simulink model "Engine_TestBench1"  (R2017a)
settings: Solver=ode1  StartTime=0.0  StopTime=1800  FixedStep=0.01  RelTol=1e-3  EnableMultiTasking=on
PostLoadFcn:
  | , if any(exist('dsrtsu_mdlpostloadfcn', 'file') == [2, 3, 6]), try dsrtsu_mdlpostloadfcn('Execute', bdroot); catch fprintf('Error in PostLoadFcn (dsrtsu_mdlpostloadfcn) for model "%s":\n %s\n', bdroot, lasterr); end, end,
undefined symbols (not defined in the file): air, Engine, env, max_vehicle_rad_air_flow, NeutralGear, ParkGear
libraries: simulink x19, EC2_libraries x2
(part 2 of 2)

== system Engine_TestBench1/ICE Simple/Engine Plant Modified/Core Engine/Crank Process/function ==
  EngSpd : Inport
  f : TriggerPort  TriggerType=function-call  VariantControl=Variant
      settings: CopyFcn=Stateflow.SLINSF.SimulinkMan.removeBlockPreDeleteFcn  PreDeleteFcn=Stateflow.SLINSF.SimulinkMan.unsafePredeleteFcn
  1-D Lookup Table : Lookup_n-D  NumberOfTableDimensions=1  BreakpointsForDimension1=[0 50 120 210 300 320 340 350 400]  Table=[90 90 90 90 90 90 90 90 90]  InternalRulePriority=Speed  RndMeth=Simplest  InputSameDT=on
  Sine Wave : Sin  Amplitude=20  Frequency=41.88
  Sum : Sum
  CrankTrq : Outport
  wires:
  1-D Lookup Table/1 -> Sum/1
  EngSpd/1 -> 1-D Lookup Table/1
  Sum/1 -> CrankTrq/1
  Sine Wave/1 -> Sum/2

== system Engine_TestBench1/ICE Simple/Engine Plant Modified/Core Engine/EngEfficiency ==
  note: Mechanical Power [W]
  Torque : Inport
  Speed : Inport  Port=2
  Fuel Consumption : Inport  Port=3
  Divide by Zero Fix : Subsystem
  Divide_by_Zero_Fix1 : EC2_libraries/Divide_by_Zero_Fix  Commented=on
  From1 : From  Commented=on  GotoTag=Wh_out
  From2 : From  Commented=on  GotoTag=Wh_in
  Goto1 : Goto  Commented=on  GotoTag=Wh_out
  Goto2 : Goto  Commented=on  GotoTag=Wh_in
  Integrator1 : Integrator  Commented=on  LimitOutput=on  LowerSaturationLimit=0
  Integrator2 : Integrator  Commented=on  LimitOutput=on  LowerSaturationLimit=0
  OnlyPositiveEnergy : Saturate  Commented=on  UpperLimit=inf  LowerLimit=0
  Percentage Efficiency : Gain  Gain=100
  Product : Product  RndMeth=Zero
  "RPM to rad/s " : Gain  Gain=pi/30
  Scope : Scope  NumInputPorts=2
  Specific Energy LHV in J/kg : Gain  Gain=Engine.Fuel.Lower_Heating_Value/1000
  Sum : Sum  Inputs=-+
  To Workspace7 : ToWorkspace  Commented=on  VariableName=eng_Wh_pos_eff_hist  SampleTime=-1
      settings: Decimation=WORKSPACE_DECIMATION
  engine_efficiency : Scope
  limit_efficiency[0-100%] : Saturate  UpperLimit=100  LowerLimit=0  ZeroCross=off
  PowerLoss : Outport
  wires:
  limit_efficiency[0-100%]/1 -> engine_efficiency/1
  Sum/1 -> PowerLoss/1  "Losses [W]"
  Fuel Consumption/1 -> Specific Energy LHV in J/kg/1
  Specific Energy LHV in J/kg/1 -> Divide by Zero Fix/2(Divide), Sum/2, Integrator2/1, Scope/2  "Thermal Power [W]"
  Torque/1 -> Product/2  "Nm"
  Speed/1 -> "RPM to rad/s "/1  "rpm"
  Percentage Efficiency/1 -> limit_efficiency[0-100%]/1  "Efficiency [%]"
  Divide by Zero Fix/1(Output) -> Percentage Efficiency/1
  Product/1 -> Scope/1, Divide by Zero Fix/1(Multiply), OnlyPositiveEnergy/1, Sum/1  "wer [W]"
  Divide_by_Zero_Fix1/1 -> To Workspace7/1
  From1/1 -> Divide_by_Zero_Fix1/1
  From2/1 -> Divide_by_Zero_Fix1/2
  Integrator1/1 -> Goto1/1
  OnlyPositiveEnergy/1 -> Integrator1/1
  Integrator2/1 -> Goto2/1
  "RPM to rad/s "/1 -> Product/1

== system Engine_TestBench1/ICE Simple/Engine Plant Modified/Core Engine/EngineThermal ==
  note: Temp Delta C deg
  PowerLoss : Inport
  Divide : Product  Inputs=*/
  Divide1 : Product  Inputs=**
  Engine Mass : Constant  Value=Engine.Mass
  Memory : Memory  X0=Engine.Init_T_amb
  Memory1 : Memory
  Product : Product  RndMeth=Zero
  Specific Heat Cap Aluminum : Constant  Value=Engine.Specific_Heat
  Sum : Sum  Inputs=|++
  Sum1 : Sum  Inputs=|+-
  tloop : Constant  Value=0.01
  Temp[degC] : Outport
  tag scope: Heat_Transfer_Eng_1=global
  wires:
  Memory1/1 -> Sum1/2
  Divide1/1 -> Divide/1  "J"
  Sum1/1 -> Divide1/2
  Memory/1 -> Sum/2
  PowerLoss/1 -> Sum1/1, [Heat_Transfer_Eng_1]  "J/s"
  Engine Mass/1 -> Product/1  "kg"
  Specific Heat Cap Aluminum/1 -> Product/2  "J/kg*K"
  Product/1 -> Divide/2
  Sum/1 -> Memory/1, Temp[degC]/1
  Divide/1 -> Sum/1
  tloop/1 -> Divide1/1
  [Heat_Reject_Eng] -> Memory1/1

== system Engine_TestBench1/ICE Simple/Engine Plant Modified/Radiator/Divide by Zero Fix ==
  Multiply : Inport
  Divide : Inport  Port=2
  Compare To Zero : simulink/Logic and Bit Operations/Compare To Zero  relop=<=  OutDataTypeStr=boolean
  Constant1 : Constant  Value=0
  Constant2 : Constant
  Product2 : Product  Inputs=/*  SaturateOnIntegerOverflow=on  InputSameDT=on  OutDataTypeStr=Inherit: Same as first input
  Switch : Switch  Threshold=1
  Switch1 : Switch  Threshold=1
  Output : Outport
  wires:
  Multiply/1 -> Product2/2
  Switch1/1 -> Output/1
  Constant1/1 -> Switch1/1
  Product2/1 -> Switch1/3
  Switch/1 -> Product2/1
  Divide/1 -> Switch/3, Compare To Zero/1
  Constant2/1 -> Switch/1
  Compare To Zero/1 -> Switch1/2, Switch/2

== system Engine_TestBench1/ICE Simple/Soft ECM/Fuel Consumption/Divide by Zero Fix ==
  Divide : Inport
  Multiply : Inport  Port=2
  Compare To Zero : simulink/Logic and Bit Operations/Compare To Zero  relop=<=  OutDataTypeStr=boolean
  Constant1 : Constant  Value=0
  Constant2 : Constant
  Product2 : Product  Inputs=/*  SaturateOnIntegerOverflow=on  InputSameDT=on  OutDataTypeStr=Inherit: Same as first input
  Switch : Switch  Threshold=1
  Switch1 : Switch  Threshold=1
  Output : Outport
  wires:
  Multiply/1 -> Product2/2
  Switch1/1 -> Output/1
  Constant1/1 -> Switch1/1
  Product2/1 -> Switch1/3
  Switch/1 -> Product2/1
  Divide/1 -> Compare To Zero/1, Switch/3
  Constant2/1 -> Switch/1
  Compare To Zero/1 -> Switch1/2, Switch/2

== system Engine_TestBench1/ICE Simple/Soft ECM/Fuel Consumption/Divide by Zero Fix1 ==
  Divide : Inport
  Multiply : Inport  Port=2
  Compare To Zero : simulink/Logic and Bit Operations/Compare To Zero  relop=<=  OutDataTypeStr=boolean
  Constant1 : Constant  Value=0
  Constant2 : Constant
  Product2 : Product  Inputs=/*  SaturateOnIntegerOverflow=on  InputSameDT=on  OutDataTypeStr=Inherit: Same as first input
  Switch : Switch  Threshold=1
  Switch1 : Switch  Threshold=1
  Output : Outport
  wires:
  Compare To Zero/1 -> Switch/2, Switch1/2
  Constant2/1 -> Switch/1
  Divide/1 -> Compare To Zero/1, Switch/3
  Switch/1 -> Product2/1
  Product2/1 -> Switch1/3
  Constant1/1 -> Switch1/1
  Switch1/1 -> Output/1
  Multiply/1 -> Product2/2

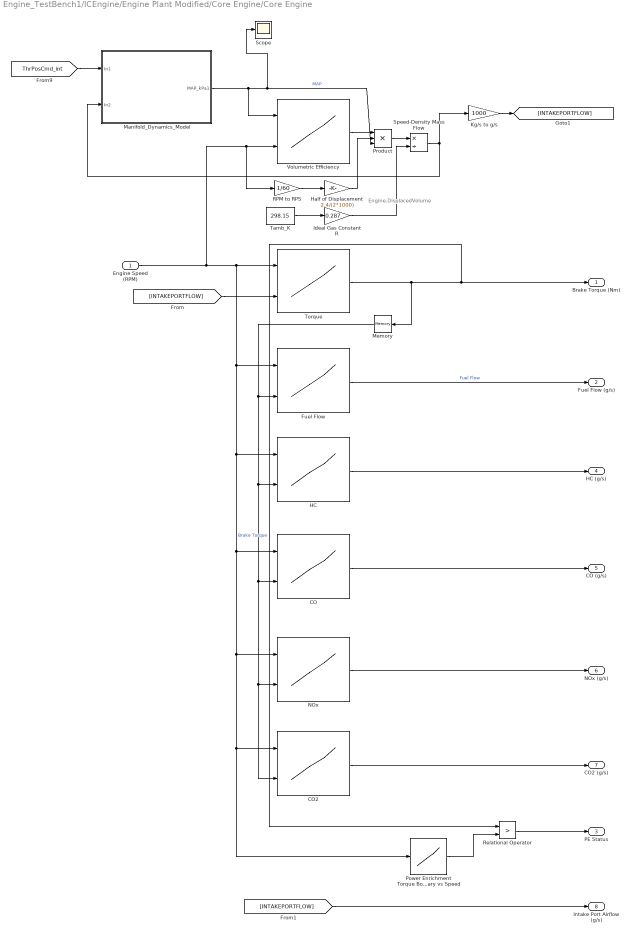
== system Engine_TestBench1/ICEngine/Engine Plant Modified/Core Engine/Core Engine ==
  note: Engine.DisplacedVolume
  Engine Speed (RPM) : Inport
  CO : Lookup2D  RowIndex=Engine.Engine.Emissions.SPEED  ColumnIndex=Engine.Engine.Emissions.TQ  Table=Engine.Engine.Emissions.CO/1000  LookUpMeth=Interpolation-Use End Values
  CO2 : Lookup2D  RowIndex=Engine.Engine.Emissions.SPEED  ColumnIndex=Engine.Engine.Emissions.TQ  Table=Engine.Engine.Emissions.CO2/1000  LookUpMeth=Interpolation-Use End Values
  Fuel Flow : Lookup2D  RowIndex=Engine.Engine.FuelFlow.SPEED  ColumnIndex=Engine.Engine.FuelFlow.TQ  Table=Engine.Engine.FuelFlow.FuelFlow  LookUpMeth=Interpolation-Use End Values
  HC : Lookup2D  RowIndex=Engine.Engine.Emissions.SPEED  ColumnIndex=Engine.Engine.Emissions.TQ  Table=Engine.Engine.Emissions.HC/1000  LookUpMeth=Interpolation-Use End Values
  Half of Displacement : Gain  Gain=2.4/(2*1000)
  Ideal Gas Constant R : Gain  Gain=0.287
  Kg/s to g/s : Gain  Gain=1000
  Manifold_Dynamics_Model : Subsystem
  Memory : Memory
  NOx : Lookup2D  RowIndex=Engine.Engine.Emissions.SPEED  ColumnIndex=Engine.Engine.Emissions.TQ  Table=Engine.Engine.Emissions.NOx/1000  LookUpMeth=Interpolation-Use End Values
  Power Enrichment Torque Boundary vs Speed : Lookup_n-D  NumberOfTableDimensions=1  BreakpointsForDimension1=Engine.Engine.PEBound.SPEED  Table=Engine.Engine.PEBound.PEBound  ExtrapMethod=Clip  InternalRulePriority=Speed  RndMeth=Simplest  InputSameDT=on
  Product : Product  Inputs=***
  RPM to RPS : Gain  Gain=1/60
  Relational Operator : RelationalOperator  Operator=>  OutDataTypeStr=boolean  RndMeth=Nearest
  Scope : Scope
  Speed-Density Mass Flow : Product  Inputs=*/
  Tamb_K : Constant  Value=298.15
  Torque : Lookup2D  RowIndex=Engine.Engine.TQ.SPEED  ColumnIndex=Engine.Engine.TQ.MAF  Table=Engine.Engine.TQ.TQ  LookUpMeth=Interpolation-Use End Values
  Volumetric Efficiency : Lookup2D  RowIndex=Engine.Engine.VE.MAP  ColumnIndex=Engine.Engine.VE.SPEED  Table=Engine.Engine.VE.VE  LookUpMeth=Interpolation-Use End Values
  Brake Torque (Nm) : Outport
  Fuel Flow (g/s) : Outport  Port=2
  PE Status : Outport  Port=3
  HC (g/s) : Outport  Port=4
  CO (g/s) : Outport  Port=5
  NOx (g/s) : Outport  Port=6
  CO2 (g/s) : Outport  Port=7
  Intake Port Airflow (g/s) : Outport  Port=8
  wires:
  Torque/1 -> Brake Torque (Nm)/1, Relational Operator/1, Memory/1  "Brake Torque"
  [INTAKEPORTFLOW] -> Torque/2
  Fuel Flow/1 -> Fuel Flow (g/s)/1  "Fuel Flow"
  Memory/1 -> CO2/2, NOx/2, CO/2, HC/2, Fuel Flow/2
  Power Enrichment Torque Boundary vs Speed/1 -> Relational Operator/2
  Relational Operator/1 -> PE Status/1
  HC/1 -> HC (g/s)/1
  CO/1 -> CO (g/s)/1
  NOx/1 -> NOx (g/s)/1
  CO2/1 -> CO2 (g/s)/1
  [INTAKEPORTFLOW] -> Intake Port Airflow (g/s)/1
  Volumetric Efficiency/1 -> Product/1
  Ideal Gas Constant R/1 -> Speed-Density Mass Flow/2
  Product/1 -> Speed-Density Mass Flow/1
  Tamb_K/1 -> Ideal Gas Constant R/1
  RPM to RPS/1 -> Half of Displacement/1
  Half of Displacement/1 -> Product/2
  Engine Speed (RPM)/1 -> Torque/1, Fuel Flow/1, HC/1, CO/1, NOx/1, Power Enrichment Torque Boundary vs Speed/1, CO2/1, RPM to RPS/1, Volumetric Efficiency/2
  [ThrPosCmd_int] -> Manifold_Dynamics_Model/1(In1)
  Manifold_Dynamics_Model/1(MAP_kPa1) -> Volumetric Efficiency/1, Scope/1, Product/3  "MAP"
  Kg/s to g/s/1 -> [INTAKEPORTFLOW]
  Speed-Density Mass Flow/1 -> Manifold_Dynamics_Model/2(In2), Kg/s to g/s/1

== system Engine_TestBench1/ICEngine/Engine Plant Modified/Core Engine/Crank Process/function ==
  EngSpd : Inport
  f : TriggerPort  TriggerType=function-call  VariantControl=Variant
      settings: CopyFcn=Stateflow.SLINSF.SimulinkMan.removeBlockPreDeleteFcn  PreDeleteFcn=Stateflow.SLINSF.SimulinkMan.unsafePredeleteFcn
  1-D Lookup Table : Lookup_n-D  NumberOfTableDimensions=1  BreakpointsForDimension1=[0 50 120 210 300 320 340 350 400]  Table=[90 90 90 90 90 90 90 90 90]  InternalRulePriority=Speed  RndMeth=Simplest  InputSameDT=on
  Sine Wave : Sin  Amplitude=20  Frequency=41.88
  Sum : Sum
  CrankTrq : Outport
  wires:
  1-D Lookup Table/1 -> Sum/1
  EngSpd/1 -> 1-D Lookup Table/1
  Sum/1 -> CrankTrq/1
  Sine Wave/1 -> Sum/2

== system Engine_TestBench1/ICEngine/Engine Plant Modified/Core Engine/EngEfficiency ==
  note: Mechanical Power [W]
  Torque : Inport
  Speed : Inport  Port=2
  Fuel Consumption : Inport  Port=3
  Divide by Zero Fix : Subsystem
  Divide_by_Zero_Fix1 : EC2_libraries/Divide_by_Zero_Fix  Commented=on
  From1 : From  Commented=on  GotoTag=Wh_out
  From2 : From  Commented=on  GotoTag=Wh_in
  Goto1 : Goto  Commented=on  GotoTag=Wh_out
  Goto2 : Goto  Commented=on  GotoTag=Wh_in
  Integrator1 : Integrator  Commented=on  LimitOutput=on  LowerSaturationLimit=0
  Integrator2 : Integrator  Commented=on  LimitOutput=on  LowerSaturationLimit=0
  OnlyPositiveEnergy : Saturate  Commented=on  UpperLimit=inf  LowerLimit=0
  Percentage Efficiency : Gain  Gain=100
  Product : Product  RndMeth=Zero
  "RPM to rad/s " : Gain  Gain=pi/30
  Scope : Scope  NumInputPorts=2
  Specific Energy LHV in J/kg : Gain  Gain=Engine.Fuel.Lower_Heating_Value/1000
  Sum : Sum  Inputs=-+
  To Workspace7 : ToWorkspace  Commented=on  VariableName=eng_Wh_pos_eff_hist  SampleTime=-1
      settings: Decimation=WORKSPACE_DECIMATION
  engine_efficiency : Scope
  limit_efficiency[0-100%] : Saturate  UpperLimit=100  LowerLimit=0
  PowerLoss : Outport
  wires:
  limit_efficiency[0-100%]/1 -> engine_efficiency/1
  Sum/1 -> PowerLoss/1  "Losses [W]"
  Fuel Consumption/1 -> Specific Energy LHV in J/kg/1
  Specific Energy LHV in J/kg/1 -> Divide by Zero Fix/2(Divide), Sum/2, Integrator2/1, Scope/2  "Thermal Power [W]"
  Torque/1 -> Product/2  "Nm"
  Speed/1 -> "RPM to rad/s "/1  "rpm"
  Percentage Efficiency/1 -> limit_efficiency[0-100%]/1  "Efficiency [%]"
  Divide by Zero Fix/1(Output) -> Percentage Efficiency/1
  Product/1 -> Scope/1, Divide by Zero Fix/1(Multiply), OnlyPositiveEnergy/1, Sum/1  "wer [W]"
  Divide_by_Zero_Fix1/1 -> To Workspace7/1
  From1/1 -> Divide_by_Zero_Fix1/1
  From2/1 -> Divide_by_Zero_Fix1/2
  Integrator1/1 -> Goto1/1
  OnlyPositiveEnergy/1 -> Integrator1/1
  Integrator2/1 -> Goto2/1
  "RPM to rad/s "/1 -> Product/1

== system Engine_TestBench1/ICEngine/Engine Plant Modified/Core Engine/EngineThermal ==
  note: Temp Delta C deg
  PowerLoss : Inport
  Divide : Product  Inputs=*/
  Divide1 : Product  Inputs=**
  Engine Mass : Constant  Value=Engine.Mass
  Memory : Memory  X0=Engine.Init_T_amb
  Memory1 : Memory
  Product : Product  RndMeth=Zero
  Specific Heat Cap Aluminum : Constant  Value=Engine.Specific_Heat
  Sum : Sum  Inputs=|++
  Sum1 : Sum  Inputs=|+-
  tloop : Constant  Value=0.01
  Temp[degC] : Outport
  tag scope: Heat_Transfer_Eng=global
  wires:
  Memory1/1 -> Sum1/2
  Divide1/1 -> Divide/1  "J"
  Sum1/1 -> Divide1/2
  Memory/1 -> Sum/2
  PowerLoss/1 -> Sum1/1, [Heat_Transfer_Eng]  "J/s"
  Engine Mass/1 -> Product/1  "kg"
  Specific Heat Cap Aluminum/1 -> Product/2  "J/kg*K"
  Product/1 -> Divide/2
  Sum/1 -> Memory/1, Temp[degC]/1
  Divide/1 -> Sum/1
  tloop/1 -> Divide1/1
  [Heat_Reject_Eng] -> Memory1/1

== system Engine_TestBench1/ICEngine/Engine Plant Modified/Radiator/Divide by Zero Fix ==
  Multiply : Inport
  Divide : Inport  Port=2
  Compare To Zero : simulink/Logic and Bit Operations/Compare To Zero  relop===  OutDataTypeStr=boolean
  Constant1 : Constant  Value=0
  Constant2 : Constant
  Product2 : Product  Inputs=/*  SaturateOnIntegerOverflow=on  InputSameDT=on  OutDataTypeStr=Inherit: Same as first input
  Switch : Switch  Threshold=1
  Switch1 : Switch  Threshold=1
  Output : Outport
  wires:
  Multiply/1 -> Product2/2
  Switch1/1 -> Output/1
  Constant1/1 -> Switch1/1
  Product2/1 -> Switch1/3
  Switch/1 -> Product2/1
  Divide/1 -> Switch/3, Compare To Zero/1
  Constant2/1 -> Switch/1
  Compare To Zero/1 -> Switch1/2, Switch/2

== system Engine_TestBench1/ICEngine/Soft ECM/Fuel Consumption/Divide by Zero Fix ==
  Divide : Inport
  Multiply : Inport  Port=2
  Compare To Zero : simulink/Logic and Bit Operations/Compare To Zero  relop===  OutDataTypeStr=boolean
  Constant1 : Constant  Value=0
  Constant2 : Constant
  Product2 : Product  Inputs=/*  SaturateOnIntegerOverflow=on  InputSameDT=on  OutDataTypeStr=Inherit: Same as first input
  Switch : Switch  Threshold=1
  Switch1 : Switch  Threshold=1
  Output : Outport
  wires:
  Multiply/1 -> Product2/2
  Switch1/1 -> Output/1
  Constant1/1 -> Switch1/1
  Product2/1 -> Switch1/3
  Switch/1 -> Product2/1
  Divide/1 -> Compare To Zero/1, Switch/3
  Constant2/1 -> Switch/1
  Compare To Zero/1 -> Switch1/2, Switch/2

== system Engine_TestBench1/ICEngine/Soft ECM/Fuel Consumption/Divide by Zero Fix1 ==
  Divide : Inport
  Multiply : Inport  Port=2
  Compare To Zero : simulink/Logic and Bit Operations/Compare To Zero  relop===  OutDataTypeStr=boolean
  Constant1 : Constant  Value=0
  Constant2 : Constant
  Product2 : Product  Inputs=/*  SaturateOnIntegerOverflow=on  InputSameDT=on  OutDataTypeStr=Inherit: Same as first input
  Switch : Switch  Threshold=1
  Switch1 : Switch  Threshold=1
  Output : Outport
  wires:
  Compare To Zero/1 -> Switch/2, Switch1/2
  Constant2/1 -> Switch/1
  Divide/1 -> Compare To Zero/1, Switch/3
  Switch/1 -> Product2/1
  Product2/1 -> Switch1/3
  Constant1/1 -> Switch1/1
  Switch1/1 -> Output/1
  Multiply/1 -> Product2/2

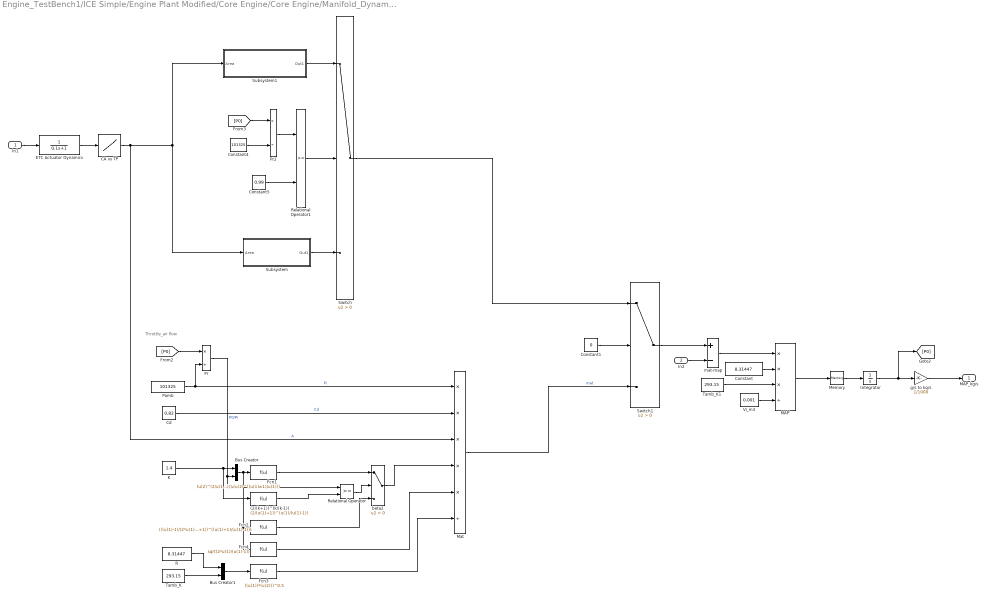
== system Engine_TestBench1/ICE Simple/Engine Plant Modified/Core Engine/Core Engine/Manifold_Dynamics_Model ==
  note: Throttle_air flow
  In1 : Inport
  In2 : Inport  Port=2
  (2/(k+1))^(k/(k-1)) : Fcn  Expr=(2/(u(1)+1))^(u(1)/(u(1)-1))
  Bus Creator : BusCreator  Inputs=2
  Bus Creator1 : BusCreator  Inputs=2
  CA vs TP : Lookup  InputValues=Engine.Throttle.CA.TPP  Table=Engine.Throttle.CA.CA  LookUpMeth=Interpolation-Use End Values
  Cd : Constant  Value=0.82
  Constant : Constant  Value=8.31447
  Constant1 : Constant  Value=0
  Constant4 : Constant  Value=101325
  Constant5 : Constant  Value=0.99
  ETC Actuator Dynamics : TransferFcn  Denominator=[0.1 1]
  Fcn1 : Fcn  Expr=(u(2)^(2/u(1)))-(u(2)^((u(1)+1)/u(1)))
  Fcn2 : Fcn  Expr=(((u(1)-1)/(2*u(1)))*(2/(u(1)+1))^((u(1)+1)/(u(1)-1)))
  Fcn3 : Fcn  Expr=((u(1))*(u(2)))^0.5
  Fcn4 : Fcn  Expr=sqrt(2*u(1)/(u(1)-1))
  Integrator : Integrator  InitialCondition=101325
  K : Constant  Value=1.4
  MAP' : Product  Inputs=***/
  Mat : Product  Inputs=*****/
  Memory : Memory
  Pamb : Constant  Value=101325
  Pr : Product  Inputs=*/
  Pr2 : Product  Inputs=*/
  R : Constant  Value=8.31447
  Relational Operator : RelationalOperator  OutDataTypeStr=boolean  ZeroCross=off  RndMeth=Nearest
  Relational Operator1 : RelationalOperator  OutDataTypeStr=boolean  ZeroCross=off  RndMeth=Nearest
  Subsystem : Subsystem
  Subsystem1 : Subsystem
  Switch : Switch  Criteria=u2 > Threshold
  Switch1 : Switch  Criteria=u2 > Threshold
  Tamb_K : Constant  Value=293.15
  Tamb_K1 : Constant  Value=293.15
  Vi_m3 : Constant  Value=0.001
  beta2 : Switch  Criteria=u2 > Threshold
  g/s to kg/s : Gain  Gain=1/1000
  mat-map : Sum  Inputs=+-
  MAP_kg/s : Outport
  wires:
  In1/1 -> ETC Actuator Dynamics/1
  Vi_m3/1 -> MAP'/4
  Constant/1 -> MAP'/2
  Tamb_K1/1 -> MAP'/3
  Switch1/1 -> mat-map/1
  In2/1 -> mat-map/2
  Integrator/1 -> g/s to kg/s/1, [P0]
  ETC Actuator Dynamics/1 -> CA vs TP/1
  Pamb/1 -> Pr/2, Mat/1  "Pi"
  Bus Creator/1 -> Fcn1/1, Fcn2/1, Fcn4/1
  Fcn3/1 -> Mat/6
  Fcn4/1 -> Mat/5
  Cd/1 -> Mat/2  "Cd"
  CA vs TP/1 -> Mat/3, Subsystem/1(Area), Subsystem1/1(Area)  "A"
  Mat/1 -> Switch1/3  "mat"
  Pr/1 -> Bus Creator/2, Relational Operator/1  "P0/Pi"
  Bus Creator1/1 -> Fcn3/1
  K/1 -> (2/(k+1))^(k/(k-1))/1, Bus Creator/1
  beta2/1 -> Mat/4
  Fcn2/1 -> beta2/3
  Fcn1/1 -> beta2/1
  R/1 -> Bus Creator1/1
  (2/(k+1))^(k/(k-1))/1 -> Relational Operator/2
  [P0] -> Pr/1
  Tamb_K/1 -> Bus Creator1/2
  Relational Operator/1 -> beta2/2
  [P0] -> Pr2/1
  Pr2/1 -> Relational Operator1/1
  Constant5/1 -> Relational Operator1/2
  Subsystem1/1(Out1) -> Switch/1
  Relational Operator1/1 -> Switch/2
  Subsystem/1(Out1) -> Switch/3
  Constant4/1 -> Pr2/2
  Switch/1 -> Switch1/1
  Constant1/1 -> Switch1/2
  MAP'/1 -> Memory/1
  Memory/1 -> Integrator/1
  mat-map/1 -> MAP'/1
  g/s to kg/s/1 -> MAP_kg/s/1

== system Engine_TestBench1/ICE Simple/Engine Plant Modified/Core Engine/EngEfficiency/Divide by Zero Fix ==
  Multiply : Inport
  Divide : Inport  Port=2
  Compare To Zero : simulink/Logic and Bit Operations/Compare To Zero  relop=<=  OutDataTypeStr=boolean
  Constant1 : Constant  Value=0
  Constant2 : Constant
  Product2 : Product  Inputs=/*  SaturateOnIntegerOverflow=on  InputSameDT=on  OutDataTypeStr=Inherit: Same as first input
  Switch : Switch  Threshold=1
  Switch1 : Switch  Threshold=1
  Output : Outport
  wires:
  Multiply/1 -> Product2/2
  Switch1/1 -> Output/1
  Constant1/1 -> Switch1/1
  Product2/1 -> Switch1/3
  Switch/1 -> Product2/1
  Divide/1 -> Switch/3, Compare To Zero/1
  Constant2/1 -> Switch/1
  Compare To Zero/1 -> Switch1/2, Switch/2

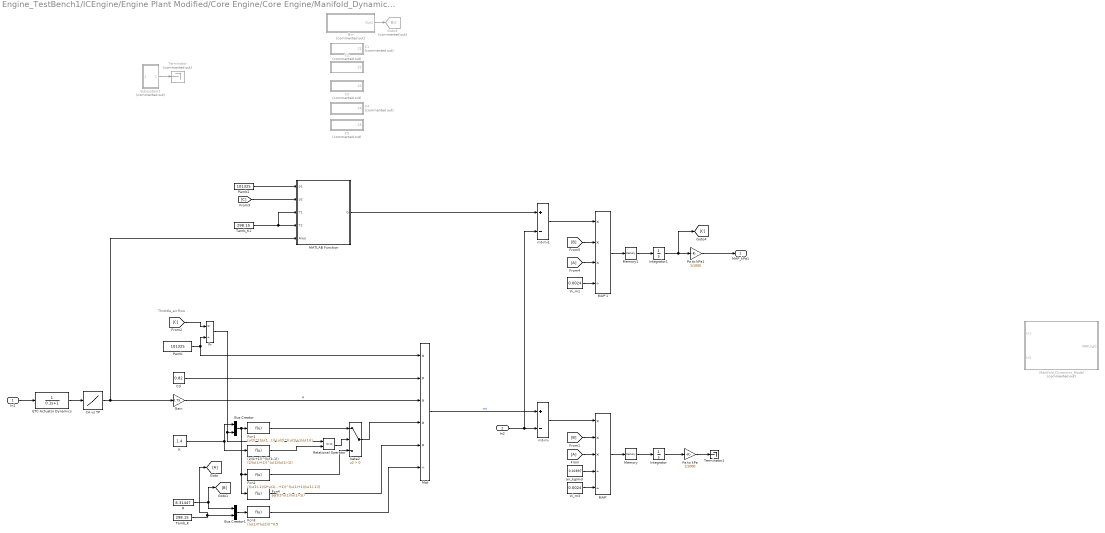
== system Engine_TestBench1/ICEngine/Engine Plant Modified/Core Engine/Core Engine/Manifold_Dynamics_Model ==
  note: Throttle_air flow
  In1 : Inport
  In2 : Inport  Port=2
  (2/(k+1))^(k/(k-1)) : Fcn  Expr=(2/(u(1)+1))^(u(1)/(u(1)-1))
  Bcr : Subsystem  Commented=on
  Bus Creator : BusCreator  Inputs=2
  Bus Creator1 : BusCreator  Inputs=2
  C1 : Subsystem  Commented=on
  C2 : Subsystem  Commented=on
  C3 : Subsystem  Commented=on
  C4 : Subsystem  Commented=on
  C5 : Subsystem  Commented=on
  CA vs TP : Lookup  InputValues=Engine.Throttle.CA.TPP  Table=Engine.Throttle.CA.CA  LookUpMeth=Interpolation-Use End Values
  Cd : Constant  Value=0.82
  ETC Actuator Dynamics : TransferFcn  Denominator=[0.1 1]
  Fcn1 : Fcn  Expr=(u(2)^(2/u(1)))-(u(2)^((u(1)+1)/u(1)))
  Fcn2 : Fcn  Expr=(((u(1)-1)/(2*u(1)))*(2/(u(1)+1))^((u(1)+1)/(u(1)-1)))
  Fcn3 : Fcn  Expr=((u(1))*(u(2)))^0.5
  Fcn4 : Fcn  Expr=sqrt(2*u(1)/(u(1)-1))
  Gain : Gain  Gain=0.75
  Goto3 : Goto  Commented=on  GotoTag=Bcr  TagVisibility=global
  Integrator : Integrator  InitialCondition=101325
  Integrator1 : Integrator  InitialCondition=101325
  K : Constant  Value=1.4
  MAP' : Product  Inputs=***//
  MAP'1 : Product  Inputs=***/
  MATLAB Function : MATLAB Function  TreatAsAtomicUnit=on
  Manifold_Dynamics_Model : Subsystem  Commented=on
  Mat : Product  Inputs=*****/
  Memory : Memory
  Memory1 : Memory
  Pa to kPa : Gain  Gain=1/1000
  Pa to kPa1 : Gain  Gain=1/1000
  Pamb : Constant  Value=101325
  Pamb1 : Constant  Value=101325
  Pr : Product  Inputs=*/
  R : Constant  Value=8.31447
  Relational Operator : RelationalOperator  OutDataTypeStr=boolean  RndMeth=Nearest
  Subsystem2 : Subsystem  Commented=on
  Tamb_K : Constant  Value=298.15
  Tamb_K1 : Constant  Value=298.15
  Terminator : Terminator  Commented=on
  Terminator1 : Terminator
  Vi_m1 : Constant  Value=0.0024
  Vi_m3 : Constant  Value=0.0024
  air_kg/mol : Constant  Value=0.02897
  beta2 : Switch  Criteria=u2 > Threshold
  mt-mi : Sum  Inputs=+-
  mt-mi1 : Sum  Inputs=+-
  MAP_kPa1 : Outport
  wires:
  In1/1 -> ETC Actuator Dynamics/1
  Mat/1 -> mt-mi/1  "mt"
  MAP'/1 -> Memory/1
  Vi_m3/1 -> MAP'/5
  [B] -> MAP'/2
  [A] -> MAP'/3
  Fcn4/1 -> Mat/5
  Tamb_K/1 -> Bus Creator1/2, [A]
  [C] -> Pr/1
  R/1 -> Bus Creator1/1, [B]
  CA vs TP/1 -> MATLAB Function/5(Area), Gain/1
  Cd/1 -> Mat/2
  Relational Operator/1 -> beta2/2
  Bus Creator1/1 -> Fcn3/1
  Pamb/1 -> Pr/2, Mat/1
  Fcn3/1 -> Mat/6
  Fcn2/1 -> beta2/3
  (2/(k+1))^(k/(k-1))/1 -> Relational Operator/2
  beta2/1 -> Mat/4
  Bus Creator/1 -> Fcn1/1, Fcn2/1, Fcn4/1
  Pr/1 -> Bus Creator/2, Relational Operator/1
  K/1 -> (2/(k+1))^(k/(k-1))/1, Bus Creator/1
  Fcn1/1 -> beta2/1
  mt-mi/1 -> MAP'/1
  In2/1 -> mt-mi1/2, mt-mi/2
  Memory/1 -> Integrator/1
  Integrator/1 -> Pa to kPa/1
  ETC Actuator Dynamics/1 -> CA vs TP/1
  Pa to kPa/1 -> Terminator1/1
  air_kg/mol/1 -> MAP'/4
  Gain/1 -> Mat/3  "A"
  Bcr/1(Out1) -> Goto3/1
  Subsystem2/1(Out1) -> Terminator/1
  [C] -> MATLAB Function/2(p2)
  Pamb1/1 -> MATLAB Function/1(p1)
  Tamb_K1/1 -> MATLAB Function/3(T1), MATLAB Function/4(T2)
  Pa to kPa1/1 -> MAP_kPa1/1
  Integrator1/1 -> [C], Pa to kPa1/1
  Memory1/1 -> Integrator1/1
  [A] -> MAP'1/3
  [B] -> MAP'1/2
  Vi_m1/1 -> MAP'1/4
  MAP'1/1 -> Memory1/1
  mt-mi1/1 -> MAP'1/1
  MATLAB Function/1(G) -> mt-mi1/1

== system Engine_TestBench1/ICEngine/Engine Plant Modified/Core Engine/EngEfficiency/Divide by Zero Fix ==
  Multiply : Inport
  Divide : Inport  Port=2
  Compare To Zero : simulink/Logic and Bit Operations/Compare To Zero  relop=<=  OutDataTypeStr=boolean
  Constant1 : Constant  Value=0
  Constant2 : Constant
  Product2 : Product  Inputs=/*  SaturateOnIntegerOverflow=on  InputSameDT=on  OutDataTypeStr=Inherit: Same as first input
  Switch : Switch  Threshold=1
  Switch1 : Switch  Threshold=1
  Output : Outport
  wires:
  Multiply/1 -> Product2/2
  Switch1/1 -> Output/1
  Constant1/1 -> Switch1/1
  Product2/1 -> Switch1/3
  Switch/1 -> Product2/1
  Divide/1 -> Switch/3, Compare To Zero/1
  Constant2/1 -> Switch/1
  Compare To Zero/1 -> Switch1/2, Switch/2

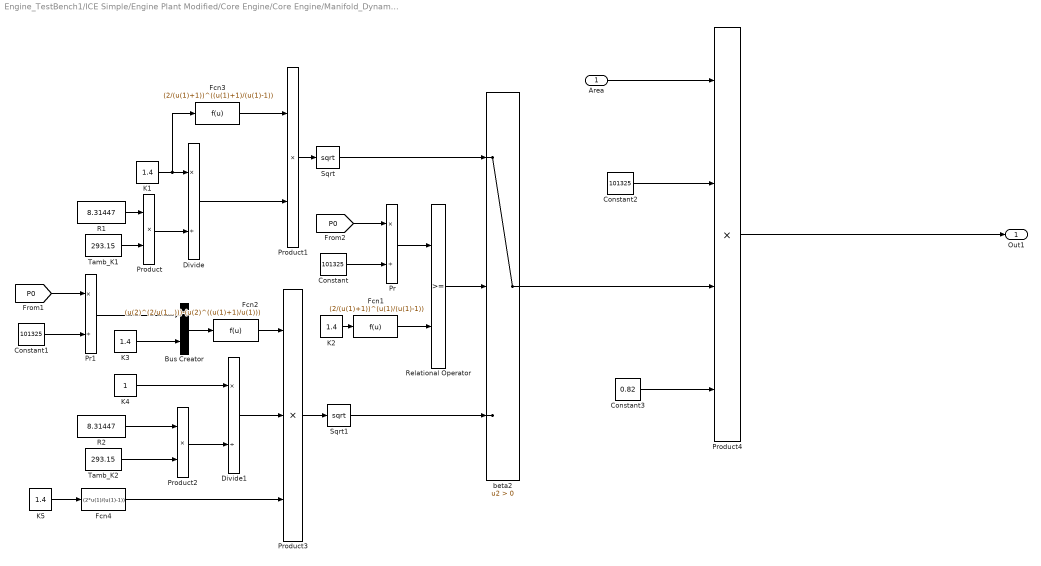
== system Engine_TestBench1/ICE Simple/Engine Plant Modified/Core Engine/Core Engine/Manifold_Dynamics_Model/Subsystem ==
  Area : Inport
  Bus Creator : BusCreator  Inputs=2
  Constant : Constant  Value=101325
  Constant1 : Constant  Value=101325
  Constant2 : Constant  Value=101325
  Constant3 : Constant  Value=0.82
  Divide : Product  Inputs=*/
  Divide1 : Product  Inputs=*/
  Fcn1 : Fcn  Expr=(2/(u(1)+1))^(u(1)/(u(1)-1))
  Fcn2 : Fcn  Expr=(u(2)^(2/u(1)))-(u(2)^((u(1)+1)/u(1)))
  Fcn3 : Fcn  Expr=(2/(u(1)+1))^((u(1)+1)/(u(1)-1))
  Fcn4 : Fcn  Expr=(2*u(1)/(u(1)-1))
  K{1..3,5} (4 alike) : Constant  Value=1.4
  K4 : Constant
  Pr : Product  Inputs=*/
  Pr1 : Product  Inputs=*/
  Product : Product
  Product1 : Product
  Product2 : Product
  Product3 : Product  Inputs=3
  Product4 : Product  Inputs=4
  R1 : Constant  Value=8.31447
  R2 : Constant  Value=8.31447
  Relational Operator : RelationalOperator  OutDataTypeStr=boolean  ZeroCross=off  RndMeth=Nearest
  Sqrt : Sqrt  SaturateOnIntegerOverflow=on
  Sqrt1 : Sqrt  SaturateOnIntegerOverflow=on
  Tamb_K1 : Constant  Value=293.15
  Tamb_K2 : Constant  Value=293.15
  beta2 : Switch  Criteria=u2 > Threshold
  Out1 : Outport
  wires:
  Product1/1 -> Sqrt/1
  Pr/1 -> Relational Operator/1
  Fcn1/1 -> Relational Operator/2
  Pr1/1 -> Bus Creator/1
  Constant1/1 -> Pr1/2
  [P0] -> Pr1/1
  Bus Creator/1 -> Fcn2/1
  K3/1 -> Bus Creator/2
  Tamb_K2/1 -> Product2/2
  K4/1 -> Divide1/1
  Product2/1 -> Divide1/2
  Divide1/1 -> Product3/2
  R2/1 -> Product2/1
  Constant/1 -> Pr/2
  Fcn3/1 -> Product1/1
  K5/1 -> Fcn4/1
  Fcn4/1 -> Product3/3
  Product4/1 -> Out1/1
  Constant2/1 -> Product4/2
  Constant3/1 -> Product4/4
  Area/1 -> Product4/1
  Sqrt/1 -> beta2/1
  [P0] -> Pr/1
  Product3/1 -> Sqrt1/1
  Fcn2/1 -> Product3/1
  beta2/1 -> Product4/3
  Tamb_K1/1 -> Product/2
  Relational Operator/1 -> beta2/2
  R1/1 -> Product/1
  Product/1 -> Divide/2
  Divide/1 -> Product1/2
  Sqrt1/1 -> beta2/3
  K2/1 -> Fcn1/1
  K1/1 -> Fcn3/1, Divide/1

== system Engine_TestBench1/ICE Simple/Engine Plant Modified/Core Engine/Core Engine/Manifold_Dynamics_Model/Subsystem1 ==
  Area : Inport
  Constant : Constant  Value=-0.5
  Constant1 : Constant  Value=0.99
  Constant2 : Constant  Value=101325
  Constant3 : Constant  Value=0.82
  Math Function : Math  Operator=pow  SaturateOnIntegerOverflow=on
  Product : Product  Inputs=5
  Subtract : Sum  Inputs=+-
  Tamb_K : Constant  Value=293.15
  Out1 : Outport
  wires:
  Constant2/1 -> Subtract/1
  Constant/1 -> Math Function/2
  Tamb_K/1 -> Math Function/1
  Constant1/1 -> Product/3
  Subtract/1 -> Product/5
  Area/1 -> Product/1
  Product/1 -> Out1/1
  Math Function/1 -> Product/4
  [P0] -> Subtract/2
  Constant3/1 -> Product/2

== system Engine_TestBench1/ICEngine/Engine Plant Modified/Core Engine/Core Engine/Manifold_Dynamics_Model/Bcr ==
  Bcr : Fcn  Expr=(2/(u(1)+1))^(u(1)/(u(1)-1))
  Constant : Constant  Value=1.4
  Out1 : Outport
  wires:
  Constant/1 -> Bcr/1
  Bcr/1 -> Out1/1

== system Engine_TestBench1/ICEngine/Engine Plant Modified/Core Engine/Core Engine/Manifold_Dynamics_Model/C1 ==
  Constant : Constant
  Divide : Product  Inputs=*/
  Gain : Gain  Gain=2
  Gain1 : Gain  Gain=8.31447
  K1 : Constant  Value=1.4
  K2 : Constant  Value=1.4
  Subtract : Sum  Inputs=+-
  C1 : Outport
  tag scope: C_1=global
  wires:
  Gain1/1 -> Divide/2
  Divide/1 -> [C_1], C1/1
  K2/1 -> Subtract/1
  K1/1 -> Gain/1
  Gain/1 -> Divide/1
  Constant/1 -> Subtract/2
  Subtract/1 -> Gain1/1

== system Engine_TestBench1/ICEngine/Engine Plant Modified/Core Engine/Core Engine/Manifold_Dynamics_Model/C2 ==
  Constant : Constant
  Divide : Product  Inputs=*/
  K1 : Constant  Value=1.4
  K2 : Constant  Value=1.4
  Subtract : Sum
  "C2 " : Outport
  tag scope: C_2=global
  wires:
  Subtract/1 -> Divide/1
  Constant/1 -> Subtract/2
  K1/1 -> Divide/2
  K2/1 -> Subtract/1
  Divide/1 -> [C_2], "C2 "/1

== system Engine_TestBench1/ICEngine/Engine Plant Modified/Core Engine/Core Engine/Manifold_Dynamics_Model/C3 ==
  Constant : Constant  Value=8.31447
  Constant1 : Constant
  Divide : Product  Inputs=**
  Divide1 : Product  Inputs=*/
  Divide2 : Product  Inputs=*/
  K2 : Constant  Value=1.4
  K3 : Constant  Value=1.4
  Math Function : Math  Operator=pow  SaturateOnIntegerOverflow=on
  Sqrt : Sqrt  SaturateOnIntegerOverflow=on
  Sum : Sum  Inputs=|++
  "C3 " : Outport
  wires:
  Divide/1 -> Sqrt/1
  K2/1 -> Divide1/1
  Constant/1 -> Divide1/2
  Divide1/1 -> Divide/1
  [Bcr] -> Math Function/1
  Constant1/1 -> Sum/1
  Sum/1 -> Divide2/1
  K3/1 -> Sum/2, Divide2/2
  Divide2/1 -> Math Function/2
  Math Function/1 -> Divide/2
  Sqrt/1 -> "C3 "/1

== system Engine_TestBench1/ICEngine/Engine Plant Modified/Core Engine/Core Engine/Manifold_Dynamics_Model/C4 ==
  Constant1 : Constant  Value=2
  Constant2 : Constant  Value=0.999
  Constant4 : Constant  Value=0.999
  Divide : Product  Inputs=**
  Divide2 : Product  Inputs=*/
  Gain : Gain  Gain=1-0.999
  K3 : Constant  Value=1.4
  Math Function : Math  Operator=pow  SaturateOnIntegerOverflow=on
  Math Function1 : Math  Operator=pow  SaturateOnIntegerOverflow=on
  Sqrt : Sqrt  SaturateOnIntegerOverflow=on
  Subtract : Sum  Inputs=+-
  "C4 " : Outport
  wires:
  Divide2/1 -> Math Function/2
  [C_1] -> Divide/1
  K3/1 -> Divide2/2
  Divide/1 -> Sqrt/1
  Constant1/1 -> Divide2/1
  Math Function/1 -> Subtract/1
  Constant2/1 -> Math Function/1
  Sqrt/1 -> Gain/1
  Constant4/1 -> Math Function1/1
  [C_2] -> Math Function1/2
  Math Function1/1 -> Subtract/2
  Subtract/1 -> Divide/2
  Gain/1 -> "C4 "/1

== system Engine_TestBench1/ICEngine/Engine Plant Modified/Core Engine/Core Engine/Manifold_Dynamics_Model/C5 ==
  Constant : Constant  Value=2/1.4
  "C5 " : Outport
  wires:
  Constant/1 -> "C5 "/1

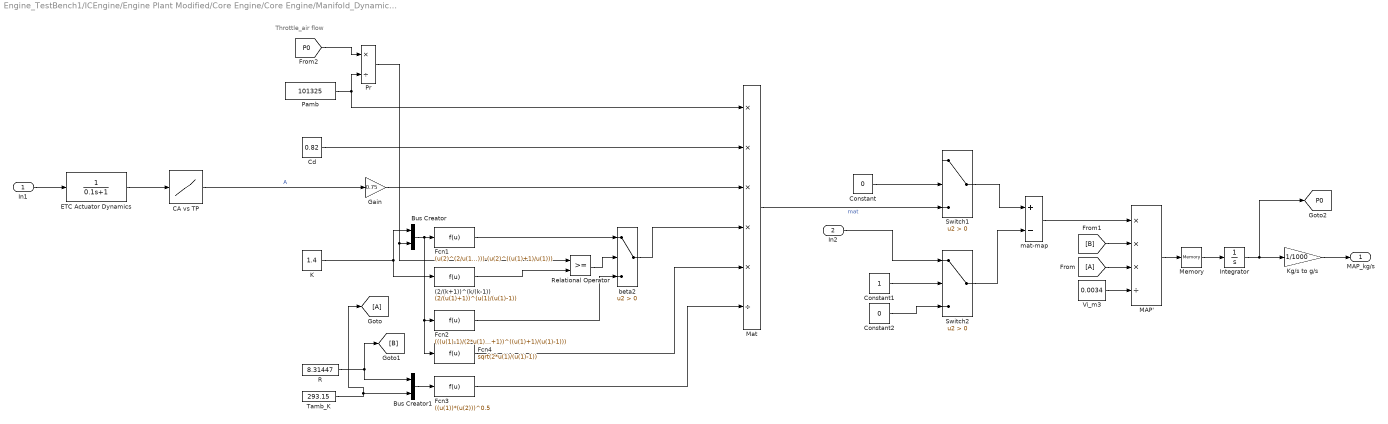
== system Engine_TestBench1/ICEngine/Engine Plant Modified/Core Engine/Core Engine/Manifold_Dynamics_Model/Manifold_Dynamics_Model ==
  note: Throttle_air flow
  In1 : Inport
  In2 : Inport  Port=2
  (2/(k+1))^(k/(k-1)) : Fcn  Expr=(2/(u(1)+1))^(u(1)/(u(1)-1))
  Bus Creator : BusCreator  Inputs=2
  Bus Creator1 : BusCreator  Inputs=2
  CA vs TP : Lookup  InputValues=Engine.Throttle.CA.TPP  Table=Engine.Throttle.CA.CA  LookUpMeth=Interpolation-Use End Values
  Cd : Constant  Value=0.82
  Constant : Constant  Value=0
  Constant1 : Constant
  Constant2 : Constant  Value=0
  ETC Actuator Dynamics : TransferFcn  Denominator=[0.1 1]
  Fcn1 : Fcn  Expr=(u(2)^(2/u(1)))-(u(2)^((u(1)+1)/u(1)))
  Fcn2 : Fcn  Expr=(((u(1)-1)/(2*u(1)))*(2/(u(1)+1))^((u(1)+1)/(u(1)-1)))
  Fcn3 : Fcn  Expr=((u(1))*(u(2)))^0.5
  Fcn4 : Fcn  Expr=sqrt(2*u(1)/(u(1)-1))
  Gain : Gain  Gain=0.75
  Integrator : Integrator  InitialCondition=101.325
  K : Constant  Value=1.4
  Kg/s to g/s : Gain  Gain=1/1000
  MAP' : Product  Inputs=***/
  Mat : Product  Inputs=*****/
  Memory : Memory
  Pamb : Constant  Value=101325
  Pr : Product  Inputs=*/
  R : Constant  Value=8.31447
  Relational Operator : RelationalOperator  OutDataTypeStr=boolean  ZeroCross=off  RndMeth=Nearest
  Switch1 : Switch  Criteria=u2 > Threshold
  Switch2 : Switch  Criteria=u2 > Threshold
  Tamb_K : Constant  Value=293.15
  Vi_m3 : Constant  Value=0.0034
  beta2 : Switch  Criteria=u2 > Threshold
  mat-map : Sum  Inputs=+-
  MAP_kg/s : Outport
  tag scope: P0=global
  wires:
  In1/1 -> ETC Actuator Dynamics/1
  Mat/1 -> Switch1/3  "mat"
  Vi_m3/1 -> MAP'/4
  [B] -> MAP'/2
  [A] -> MAP'/3
  Fcn4/1 -> Mat/5
  Tamb_K/1 -> Bus Creator1/2, [A]
  [P0] -> Pr/1
  R/1 -> Bus Creator1/1, [B]
  Cd/1 -> Mat/2
  Relational Operator/1 -> beta2/2
  Bus Creator1/1 -> Fcn3/1
  Pamb/1 -> Pr/2, Mat/1
  Fcn3/1 -> Mat/6
  Fcn2/1 -> beta2/3
  (2/(k+1))^(k/(k-1))/1 -> Relational Operator/2
  beta2/1 -> Mat/4
  Bus Creator/1 -> Fcn1/1, Fcn2/1, Fcn4/1
  Pr/1 -> Bus Creator/2, Relational Operator/1
  K/1 -> Bus Creator/1, (2/(k+1))^(k/(k-1))/1
  Fcn1/1 -> beta2/1
  mat-map/1 -> MAP'/1
  In2/1 -> Switch2/1
  ETC Actuator Dynamics/1 -> CA vs TP/1
  Gain/1 -> Mat/3
  CA vs TP/1 -> Gain/1  "A"
  Switch1/1 -> mat-map/1
  Constant/1 -> Switch1/2
  MAP'/1 -> Memory/1
  Constant1/1 -> Switch2/2
  Constant2/1 -> Switch2/3
  Switch2/1 -> mat-map/2
  Integrator/1 -> Kg/s to g/s/1, [P0]
  Kg/s to g/s/1 -> MAP_kg/s/1
  Memory/1 -> Integrator/1

== system Engine_TestBench1/ICEngine/Engine Plant Modified/Core Engine/Core Engine/Manifold_Dynamics_Model/Subsystem2 ==
  In1 : Inport
  Constant4 : Constant  Value=101325
  Constant5 : Constant  Value=0.99
  Pr2 : Product  Inputs=*/
  Relational Operator1 : RelationalOperator  Operator=>  OutDataTypeStr=boolean  ZeroCross=off  RndMeth=Nearest
  Subsystem : Subsystem
  Subsystem1 : Subsystem
  Switch : Switch  Criteria=u2 > Threshold
  Out1 : Outport
  wires:
  Pr2/1 -> Relational Operator1/1
  Subsystem/1(Out1) -> Switch/3
  Constant5/1 -> Relational Operator1/2
  Constant4/1 -> Pr2/2
  Subsystem1/1(Out1) -> Switch/1
  [C] -> Pr2/1
  Relational Operator1/1 -> Switch/2
  Switch/1 -> Out1/1
  In1/1 -> Subsystem/1(Area), Subsystem1/1(Area)

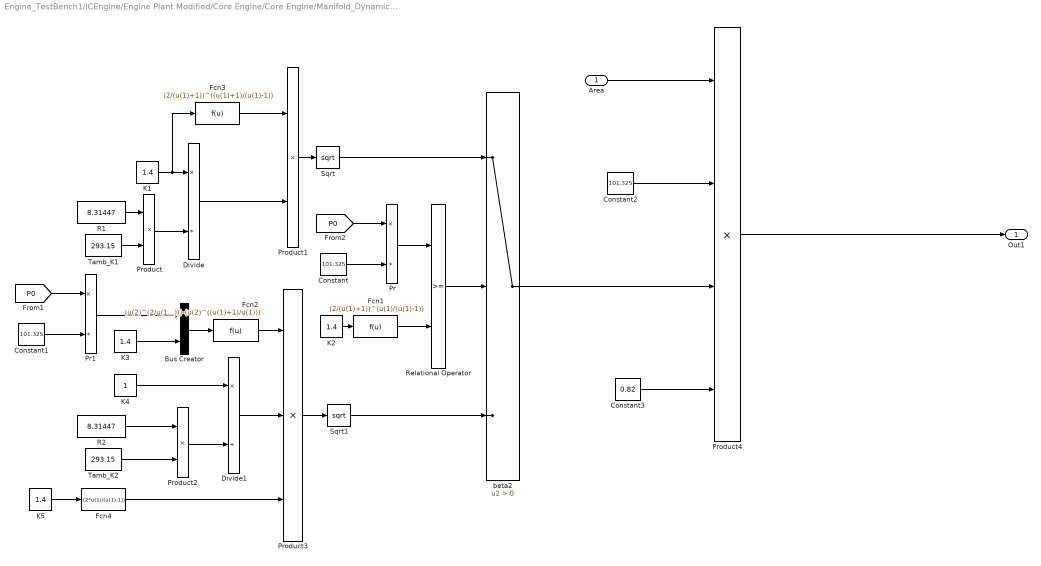
== system Engine_TestBench1/ICEngine/Engine Plant Modified/Core Engine/Core Engine/Manifold_Dynamics_Model/Subsystem2/Subsystem ==
  Area : Inport
  Bus Creator : BusCreator  Inputs=2
  Constant : Constant  Value=101.325
  Constant1 : Constant  Value=101.325
  Constant2 : Constant  Value=101.325
  Constant3 : Constant  Value=0.82
  Divide : Product  Inputs=*/
  Divide1 : Product  Inputs=*/
  Fcn1 : Fcn  Expr=(2/(u(1)+1))^(u(1)/(u(1)-1))
  Fcn2 : Fcn  Expr=(u(2)^(2/u(1)))-(u(2)^((u(1)+1)/u(1)))
  Fcn3 : Fcn  Expr=(2/(u(1)+1))^((u(1)+1)/(u(1)-1))
  Fcn4 : Fcn  Expr=(2*u(1)/(u(1)-1))
  K{1..3,5} (4 alike) : Constant  Value=1.4
  K4 : Constant
  Pr : Product  Inputs=*/
  Pr1 : Product  Inputs=*/
  Product : Product
  Product1 : Product
  Product2 : Product
  Product3 : Product  Inputs=3
  Product4 : Product  Inputs=4
  R1 : Constant  Value=8.31447
  R2 : Constant  Value=8.31447
  Relational Operator : RelationalOperator  OutDataTypeStr=boolean  ZeroCross=off  RndMeth=Nearest
  Sqrt : Sqrt  SaturateOnIntegerOverflow=on
  Sqrt1 : Sqrt  SaturateOnIntegerOverflow=on
  Tamb_K1 : Constant  Value=293.15
  Tamb_K2 : Constant  Value=293.15
  beta2 : Switch  Criteria=u2 > Threshold
  Out1 : Outport
  wires:
  Product1/1 -> Sqrt/1
  Pr/1 -> Relational Operator/1
  Fcn1/1 -> Relational Operator/2
  Pr1/1 -> Bus Creator/1
  Constant1/1 -> Pr1/2
  [P0] -> Pr1/1
  Bus Creator/1 -> Fcn2/1
  K3/1 -> Bus Creator/2
  Tamb_K2/1 -> Product2/2
  K4/1 -> Divide1/1
  Product2/1 -> Divide1/2
  Divide1/1 -> Product3/2
  R2/1 -> Product2/1
  Constant/1 -> Pr/2
  Fcn3/1 -> Product1/1
  K5/1 -> Fcn4/1
  Fcn4/1 -> Product3/3
  Product4/1 -> Out1/1
  Constant2/1 -> Product4/2
  Constant3/1 -> Product4/4
  Area/1 -> Product4/1
  Sqrt/1 -> beta2/1
  [P0] -> Pr/1
  Product3/1 -> Sqrt1/1
  Fcn2/1 -> Product3/1
  beta2/1 -> Product4/3
  Tamb_K1/1 -> Product/2
  Relational Operator/1 -> beta2/2
  R1/1 -> Product/1
  Product/1 -> Divide/2
  Divide/1 -> Product1/2
  Sqrt1/1 -> beta2/3
  K2/1 -> Fcn1/1
  K1/1 -> Fcn3/1, Divide/1

== system Engine_TestBench1/ICEngine/Engine Plant Modified/Core Engine/Core Engine/Manifold_Dynamics_Model/Subsystem2/Subsystem1 ==
  Area : Inport
  Constant : Constant  Value=-0.5
  Constant1 : Constant  Value=0.99
  Constant2 : Constant  Value=101325
  Constant3 : Constant  Value=0.82
  Math Function : Math  Operator=pow  SaturateOnIntegerOverflow=on
  Product : Product  Inputs=5
  Subtract : Sum  Inputs=+-
  Tamb_K : Constant  Value=293.15
  Out1 : Outport
  wires:
  Constant2/1 -> Subtract/1
  Constant/1 -> Math Function/2
  Tamb_K/1 -> Math Function/1
  Constant1/1 -> Product/3
  Subtract/1 -> Product/5
  Area/1 -> Product/1
  Product/1 -> Out1/1
  Math Function/1 -> Product/4
  [P0] -> Subtract/2
  Constant3/1 -> Product/2

== matlab function Engine_TestBench1/ICEngine/Engine Plant Modified/Core Engine/Core Engine/Manifold_Dynamics_Model/MATLAB Function ==
  data: p1 input; G output; p2 input; T1 input; T2 input; Area input
function G = fcn(p1,p2,T1,T2,Area)
Cd    = 0.82;    % Discharge coefficient, Cd
Area0 = 1e-12; % Minimum area'm^2'
Bcr = 0.5283;    % Critical pressure ratio (for choked flow)'1'
Blam  = 0.999;    % Pressure ratio above which a linear solution is used '1'
p_min = 0.01;    % Minimum absolute pressure expected in simulation  'Pa'
T_min = 0.01;     % Minimum absolute temperature expected in simulation, 'K'
p_gradient_min = 100;% 1/p_min
T_gradient_min = 100;   % 1/T_min
p_offset_min = log(0.01); % log(p_min) , '1'
T_offset_min = log(0.01); % log(T_min)'1'
T_unit = 1;        % Units of temperature , 'K'
p_unit = 1;       % Units of pressure , 'Pa'
c_p = 1005 ;        % Specific heat at constant pressure, 'J/kg/K' 
c_v = 717.95 ;      % Specific heat at constant volume, 'J/kg/K' 
gam = c_p/c_v; %Specific heat of air
R = 8.31447; %Ideal Gas Constant

% Calculate critical pressure ratio
Bcr = (2/(gam+1))^(gam/(gam-1));
% Calculate collected constant terms for flow equation
c_1 = 2*gam/(R*(gam-1));
c_2 = (gam+1)/gam;
c_3 = sqrt( (gam/R)*Bcr^((gam+1)/gam) );
c_4 = sqrt( c_1 * ( Blam^(2/gam) - Blam^c_2 ) ) / (1-Blam);
c_5 = 2/gam;


if lt(p1,p_min)
    logP1 =  p_offset_min + p_gradient_min*(p1 - p_min);
else
    logP1 = log(p1/p_unit);
end
if lt(p2,p_min)
    logP2 =  p_offset_min + p_gradient_min*(p2 - p_min);
else
    logP2 = log(p2/p_unit) ;
end
if lt(T1,T_min)
    logT1 =  T_offset_min + T_gradient_min*(T1 - T_min);
else
    logT1 = log(T1/T_unit);
end
if lt(T2,T_min)
    logT2 =  T_offset_min + T_gradient_min*(T2 - T_min) ;
else
    logT2 = log(T2/T_unit);
end

% Flow direction - "dir" is positive if flow is from port A to port B, otherwise negative.
if ge(p1,p2)
    dir = 1;
else
    dir = -1;
end

% Upstream and downstream pressures and temperatures
if ge(p1,p2)
    p_u = p_unit*exp(logP1);
    p_d = p_unit*exp(logP2);
    T_u = T_unit*exp(logT1);
    T_d = T_unit*exp(logT2);
else
    p_u = p_unit*exp(logP2);
    p_d = p_unit*exp(logP1);
    T_u = T_unit*exp(logT2);
    T_d = T_unit*exp(logT1);
end

% Area - limit to be greater than Area0
if Area < Area0
    AreaL = Area0;
else
    AreaL =  Area;
end
if gt(p_d/p_u, Blam)    % Laminar flow
    G = dir*Cd*AreaL*c_4*(p_u-p_d)/sqrt(T_u);
elseif gt(p_d/p_u, Bcr) % Subsonic flow
    G = dir*Cd*AreaL*p_u*sqrt( c_1 * ( (p_d/p_u)^c_5 - (p_d/p_u)^c_2) )/sqrt(T_u);
else                 % Choked flow
    G = dir*Cd*AreaL*p_u*c_3 / sqrt(T_u);
end
end

== stateflow chart Engine_TestBench1/ICE Simple/Engine Plant Modified/Core Engine/Crank Process ==
  state Starter_Crank
    du:
    EngActTrq = function(EngSpd_RPM);
  state Eng_Off
    du:
    EngActTrq = 0;
  state Eng_Combustion
    du:
    EngActTrq = 100;
  state CrankTrq = function(EngSpd) [function]
  state Eng_Run
    du:
    EngActTrq = EngBrkTrq;
  (default) -> Eng_Off
  Eng_Off -> Starter_Crank : [EngCrankCmd]
  Starter_Crank -> Eng_Off [order 2] : [!EngCrankCmd]
  Eng_Run -> Eng_Off : [AvlblFuel <= 0.01|| EngShutdown == 1]
  Starter_Crank -> Eng_Combustion [order 1] : [AvlblFuel >= 0.1]
  Eng_Combustion -> Eng_Run : [EngRunAtv]
  data: CrankTrq function_output; EngSpd function_input; EngRunAtv input boolean; AvlblFuel input double; EngActTrq output double; EngCrankCmd input boolean; EngBrkTrq input double; EngSpd_RPM input double; EngShutdown input boolean

== stateflow chart Engine_TestBench1/ICE Simple/Soft ECM/ECM_RollingAliveCnt/Rolling Alive Counter ==
  state RollingAliveCounter
    state Count1
      en: RollingAliveCnt = 0;
    state Count2
      en: RollingAliveCnt = 1;
    state Count3
      en: RollingAliveCnt = 2;
    state Count4
      en: RollingAliveCnt = 3;
    (default) -> Count1
    Count4 -> Count1 : after(0.01,sec)
    Count1 -> Count2 : after(0.01,sec)
    Count2 -> Count3 : after(0.01,sec)
    Count3 -> Count4 : after(0.01,sec)
  data: RollingAliveCnt output int8 =0

== stateflow chart Engine_TestBench1/ICE Simple/Soft ECM/Logic ==
  state Eng_Off
    en:
    EngRunAtv = 0;
    EngCrankCmd = 0;
    FuelPumpEnable = 0;
    du:
    ThrottleCmd = APP2TP(EngSpd_RPM,drvAPP,ShftLvrPos);
  state Eng_Crank
    en:
    EngCrankCmd = 1;
    FuelPumpEnable = 1;
    EngShutdown = 0;
  state Eng_On
    en:
    EngRunAtv = 1;
    EngCrankCmd = 0;
    du:
    ThrottleCmd = APP2TP(EngSpd_RPM,drvAPP,ShftLvrPos);
  state TP = APP2TP(EngSpd,APP,Shifter) [function]
  (default) -> Eng_Off
  Eng_Off -> Eng_Crank : [SysPwrMd == 3]
  Eng_Crank -> Eng_Off [order 2] : [SysPwrMd < 3]
  Eng_Crank -> Eng_On [order 1] : [EngSpd_RPM >= 580]
  Eng_On -> Eng_Off : [SysPwrMd < 2 || EngSpd_RPM < 500]
      | {EngShutdown = 1; }
  data: EngSpd function_input; TP function_output; APP function_input; Shifter function_input; drvAPP input; ThrottleCmd output double; EngCrankCmd output boolean; SysPwrMd input int8; ShftLvrPos input int8; EngSpd_RPM input double; VehSpdAvgDrvn input double; EngRunAtv output boolean; FuelPumpEnable output double; EngShutdown output boolean

== stateflow chart Engine_TestBench1/ICEngine/Engine Plant Modified/Core Engine/Crank Process ==
  state Starter_Crank
    du:
    EngActTrq = function(EngSpd_RPM);
  state Eng_Off
    du:
    EngActTrq = 0;
  state Eng_Combustion
    du:
    EngActTrq = 100;
  state CrankTrq = function(EngSpd) [function]
  state Eng_Run
    du:
    EngActTrq = EngBrkTrq;
  (default) -> Eng_Off
  Eng_Off -> Starter_Crank : [EngCrankCmd]
  Starter_Crank -> Eng_Off [order 2] : [!EngCrankCmd]
  Eng_Run -> Eng_Off : [AvlblFuel <= 0.01|| EngShutdown == 1]
  Starter_Crank -> Eng_Combustion [order 1] : [AvlblFuel >= 0.1]
  Eng_Combustion -> Eng_Run : [EngRunAtv]
  data: CrankTrq function_output; EngSpd function_input; EngRunAtv input boolean; AvlblFuel input double; EngActTrq output double; EngCrankCmd input boolean; EngBrkTrq input double; EngSpd_RPM input double; EngShutdown input boolean

== stateflow chart Engine_TestBench1/ICEngine/Soft ECM/ECM_RollingAliveCnt/Rolling Alive Counter ==
  state RollingAliveCounter
    state Count1
      en: RollingAliveCnt = 0;
    state Count2
      en: RollingAliveCnt = 1;
    state Count3
      en: RollingAliveCnt = 2;
    state Count4
      en: RollingAliveCnt = 3;
    (default) -> Count1
    Count4 -> Count1 : after(0.01,sec)
    Count1 -> Count2 : after(0.01,sec)
    Count2 -> Count3 : after(0.01,sec)
    Count3 -> Count4 : after(0.01,sec)
  data: RollingAliveCnt output int8 =0

== stateflow chart Engine_TestBench1/ICEngine/Soft ECM/Logic ==
  state Eng_Crank
    en:
    EngCrankCmd = 1;
    FuelPumpEnable = 1;
    EngShutdown = 0;
  state Eng_Off
    en:
    EngRunAtv = 0;
    EngCrankCmd = 0;
    ThrottleCmd = 0;
    FuelPumpEnable = 0;
  state Eng_On
    en:
    EngRunAtv = 1;
    EngCrankCmd = 0;
    du:
    ThrottleCmd = APP2TP(EngSpd_RPM,drvAPP,ShftLvrPos);
  state TP = APP2TP(EngSpd,APP,Shifter) [function]
  (default) -> Eng_Off
  Eng_Off -> Eng_Crank : [SysPwrMd == 3]
  Eng_Crank -> Eng_Off [order 2] : [SysPwrMd < 3]
  Eng_On -> Eng_Off : [SysPwrMd < 2 || EngSpd_RPM < 500]
      | {EngShutdown = 1; }
  Eng_Crank -> Eng_On [order 1] : [EngSpd_RPM >= 580]
  data: EngSpd function_input; TP function_output; APP function_input; Shifter function_input; drvAPP input; ThrottleCmd output double; EngCrankCmd output boolean; SysPwrMd input int8; ShftLvrPos input int8; EngSpd_RPM input double; VehSpdAvgDrvn input double; EngRunAtv output boolean; FuelPumpEnable output double; EngShutdown output boolean
